simulink model "TCPrt_TrqLim"  (R2016b)
settings: configuration reference "CodeGenConfigSet" (kept outside this file)
values from neighbouring files (symbols this model uses):
  TCPrt_nSpdMax_CUR = Calibration.Parameter    [init_TCPrt_TrqLim.m]    (also in init_TCPrt_TrqLim_SIL.m = Simulink.Parameter)
  TCPrt_nSpdMax_CURX = Calibration.Parameter    [init_TCPrt_TrqLim.m]    (also in init_TCPrt_TrqLim_SIL.m = Simulink.Parameter)
  TCPrt_tiOvrSpdDebDef_C = Calibration.Parameter    [init_TCPrt_TrqLim.m]    (also in init_TCPrt_TrqLim_SIL.m = Simulink.Parameter)
  TCPrt_tiOvrSpdDebOk_C = Calibration.Parameter    [init_TCPrt_TrqLim.m]    (also in init_TCPrt_TrqLim_SIL.m = Simulink.Parameter)
  TCPrt_trqMax_CUR = Calibration.Parameter    [init_TCPrt_TrqLim.m]    (also in init_TCPrt_TrqLim_SIL.m = Simulink.Parameter)
  TCPrt_trqMax_CURX = Calibration.Parameter    [init_TCPrt_TrqLim.m]    (also in init_TCPrt_TrqLim_SIL.m = Simulink.Parameter)
  TCPrt_trqOpnLop_MAP = Calibration.Parameter    [init_TCPrt_TrqLim.m]    (also in init_TCPrt_TrqLim_SIL.m = Simulink.Parameter)
  TCPrt_trqOpnLop_MAPX = Calibration.Parameter    [init_TCPrt_TrqLim.m]    (also in init_TCPrt_TrqLim_SIL.m = Simulink.Parameter)
  TCPrt_trqOpnLop_MAPY = Calibration.Parameter    [init_TCPrt_TrqLim.m]    (also in init_TCPrt_TrqLim_SIL.m = Simulink.Parameter)
  TRQ_MAX = fi(1000,Trq_Nm)    [init_TCPrt_TrqLim.m]    (also in init_TCPrt_TrqLim_SIL.m)
undefined symbols (not defined in the file or in its folder): CEngDsT_tTransf_CURX, TCPrt_TrqLim_DT
libraries: CXLib x3
settings Model: Creator=GaberXu  LastModifiedBy=wangrui
settings ConfigSetRef: SourceLocation=Base Workspace

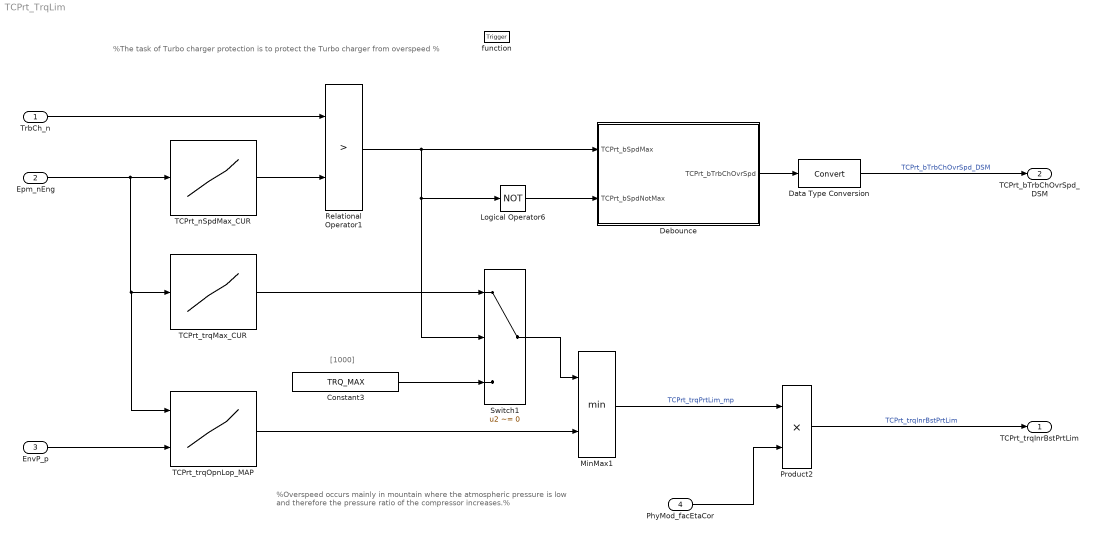
== system TCPrt_TrqLim ==
  note: [1000]
  note: %Overspeed occurs mainly in mountain where the atmospheric pressure is low and therefore the pressure ratio of the compressor increases.%
  note: %The task of Turbo charger protection is to protect the Turbo charger from overspeed %
  TrbCh_n : Inport  Tag=rpm  Description=Turbo charger speed  OutMin=-327679  OutMax=327671  OutDataTypeStr=Turbo_rpm
  Epm_nEng : Inport  Tag=rpm  Description=Engine speed  Port=2  OutMin=0  OutMax=6000  OutDataTypeStr=EngSpeed_rpm
  EnvP_p : Inport  Tag=kPa  Description=Barometric pressure  Port=3  OutMin=0  OutMax=3276  OutDataTypeStr=AirPressure_kPa
  PhyMod_facEtaCor : Inport  Description=Current efficiency correction factor  Port=4  OutMin=-30  OutMax=30  OutDataTypeStr=Factor
  function : TriggerPort  TriggerType=function-call  VariantControl=Variant
  Constant3 : Constant  RequirementInfo={'other' 'APP_requirements.doc' '@Simulink_requirement_item_25' 'true' '手动开关' '' } %GIDa_ac8829b9_b6f4_4cbb_b4cf_837d8217a02f  Value=TRQ_MAX  OutDataTypeStr=Inherit: Inherit via back propagation  SampleTime=-1
  Data Type Conversion : DataTypeConversion
  Debounce : Subsystem
  Logical Operator6 : Logic  Operator=NOT  AllPortsSameDT=off  OutDataTypeStr=boolean
  MinMax1 : MinMax  Inputs=2  SaturateOnIntegerOverflow=on  InputSameDT=on
  Product2 : Product  OutDataTypeStr=Inherit: Inherit via back propagation  SaturateOnIntegerOverflow=on
  Relational Operator1 : RelationalOperator  Operator=>  OutDataTypeStr=boolean  RndMeth=Simplest  InputSameDT=on
  Switch1 : Switch  Criteria=u2 ~= 0  SaturateOnIntegerOverflow=on  InputSameDT=on
  TCPrt_nSpdMax_CUR : Lookup_n-D  RequirementInfo={} %GIDa_17a547b7_83b2_4217_9b4d_3a7f90d79b37  DialogController=Simulink.DDGSource  NumberOfTableDimensions=1  BreakpointsForDimension1=TCPrt_nSpdMax_CURX  BreakpointsForDimension2=CEngDsT_tTransf_CURX  IndexSearchMethod=Linear search  BeginIndexSearchUsingPreviousIndexResult=on  Table=TCPrt_nSpdMax_CUR  ExtrapMethod=Clip  UseLastTableValue=on  InternalRulePriority=Speed  OutDataTypeStr=Inherit: Inherit via back propagation  SaturateOnIntegerOverflow=on
  TCPrt_trqMax_CUR : Lookup_n-D  RequirementInfo={} %GIDa_8e7e3ec2_6cdf_493c_bf9f_71de08a6e3ac  DialogController=Simulink.DDGSource  NumberOfTableDimensions=1  BreakpointsForDimension1=TCPrt_trqMax_CURX  BreakpointsForDimension2=CEngDsT_tTransf_CURX  IndexSearchMethod=Linear search  BeginIndexSearchUsingPreviousIndexResult=on  Table=TCPrt_trqMax_CUR  ExtrapMethod=Clip  UseLastTableValue=on  InternalRulePriority=Speed  OutDataTypeStr=Inherit: Inherit via back propagation  SaturateOnIntegerOverflow=on
  TCPrt_trqOpnLop_MAP : Lookup_n-D  RequirementInfo={} %GIDa_14388a41_a816_4e07_ba4a_17d21c99ac02  DialogController=Simulink.DDGSource  BreakpointsForDimension1=TCPrt_trqOpnLop_MAPY  BreakpointsForDimension2=TCPrt_trqOpnLop_MAPX  IndexSearchMethod=Linear search  BeginIndexSearchUsingPreviousIndexResult=on  Table=TCPrt_trqOpnLop_MAP  ExtrapMethod=Clip  UseLastTableValue=on  InternalRulePriority=Speed  OutDataTypeStr=Inherit: Inherit via back propagation  SaturateOnIntegerOverflow=on
  TCPrt_trqInrBstPrtLim : Outport  Tag=Nm  Description=Torque limitation from VGT Nm  OutMin=-3276.8  OutMax=3276.7  OutDataTypeStr=Trq_Nm
  TCPrt_bTrbChOvrSpd_DSM : Outport  Description=Turbine overspeed fault(output to DSM)  Port=2  OutMin=0  OutMax=1  OutDataTypeStr=boolean
  wires:
  Product2/1 -> TCPrt_trqInrBstPrtLim/1  "TCPrt_trqInrBstPrtLim"
  Logical Operator6/1 -> Debounce/2(TCPrt_bSpdNotMax)
  TCPrt_trqMax_CUR/1 -> Switch1/1
  EnvP_p/1 -> TCPrt_trqOpnLop_MAP/2
  Epm_nEng/1 -> TCPrt_trqOpnLop_MAP/1, TCPrt_trqMax_CUR/1, TCPrt_nSpdMax_CUR/1
  TrbCh_n/1 -> Relational Operator1/1
  Constant3/1 -> Switch1/3
  MinMax1/1 -> Product2/1  "TCPrt_trqPrtLim_mp"
  Debounce/1(TCPrt_bTrbChOvrSpd) -> Data Type Conversion/1
  Relational Operator1/1 -> Logical Operator6/1, Switch1/2, Debounce/1(TCPrt_bSpdMax)
  TCPrt_nSpdMax_CUR/1 -> Relational Operator1/2
  TCPrt_trqOpnLop_MAP/1 -> MinMax1/2
  Switch1/1 -> MinMax1/1
  PhyMod_facEtaCor/1 -> Product2/2
  Data Type Conversion/1 -> TCPrt_bTrbChOvrSpd_DSM/1  "TCPrt_bTrbChOvrSpd_DSM"

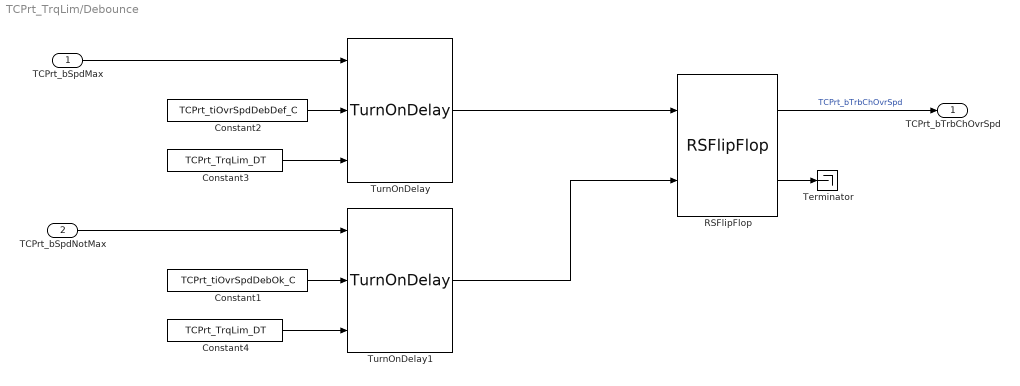
== system TCPrt_TrqLim/Debounce ==
  TCPrt_bSpdMax : Inport
  TCPrt_bSpdNotMax : Inport  Port=2
  Constant1 : Constant  Value=TCPrt_tiOvrSpdDebOk_C
  Constant2 : Constant  Value=TCPrt_tiOvrSpdDebDef_C
  Constant3 : Constant  Value=TCPrt_TrqLim_DT
  Constant4 : Constant  Value=TCPrt_TrqLim_DT
  RSFlipFlop : CXLib/RSFlipFlop
  Terminator : Terminator
  TurnOnDelay : CXLib/TurnOnDelay
  TurnOnDelay1 : CXLib/TurnOnDelay
  TCPrt_bTrbChOvrSpd : Outport
  wires:
  Constant4/1 -> TurnOnDelay1/3
  Constant3/1 -> TurnOnDelay/3
  TCPrt_bSpdMax/1 -> TurnOnDelay/1
  RSFlipFlop/2 -> Terminator/1
  TCPrt_bSpdNotMax/1 -> TurnOnDelay1/1
  TurnOnDelay/1 -> RSFlipFlop/1
  Constant2/1 -> TurnOnDelay/2
  Constant1/1 -> TurnOnDelay1/2
  TurnOnDelay1/1 -> RSFlipFlop/2
  RSFlipFlop/1 -> TCPrt_bTrbChOvrSpd/1  "TCPrt_bTrbChOvrSpd"
